simulink model "E11_implementation"  (R2017a)
settings: Solver=VariableStepAuto  StartTime=0.0  StopTime=100  RelTol=1e-3
InitFcn:
  | clear
  | E_param
undefined symbols (not defined in the file or in its folder): E_animation
settings Model: Creator=Mat Haskell  LastModifiedBy=Mat Haskell

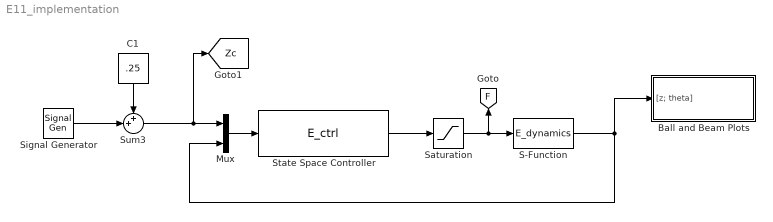
== system E11_implementation ==
  Ball and Beam Plots : Subsystem
  C1 : Constant  Value=.25
  Mux : Mux  Inputs=2
  S-Function : S-Function  FunctionName=E_dynamics  Parameters=P  SFunctionDeploymentMode=off  EnableBusSupport=off
  Saturation : Saturate  UpperLimit=15  LowerLimit=0
  Signal Generator : SignalGenerator  WaveForm=square  Amplitude=.125  Frequency=.05
  State Space Controller : MATLABFcn  MATLABFcn=E_ctrl
  Sum3 : Sum  Inputs=++|
  tag scope: F=global, Zc=global
  wires:
  Sum3/1 -> [Zc], Mux/1
  Saturation/1 -> S-Function/1, [F]
  S-Function/1 -> Mux/2, Ball and Beam Plots/1("[z; theta]")
  C1/1 -> Sum3/1
  Signal Generator/1 -> Sum3/2
  State Space Controller/1 -> Saturation/1
  Mux/1 -> State Space Controller/1

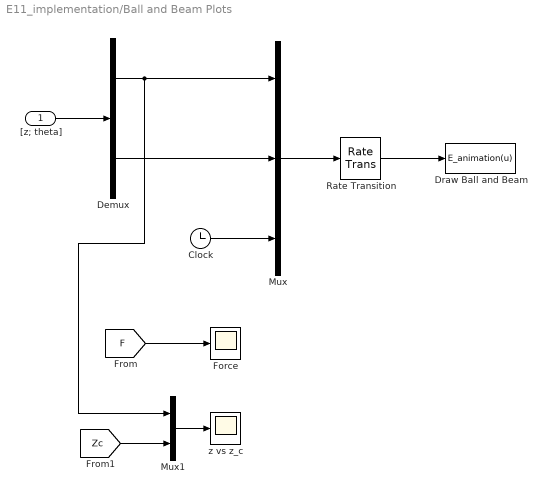
== system E11_implementation/Ball and Beam Plots ==
  "[z; theta]" : Inport
  Clock : Clock
  Demux : Demux  Outputs=2
  Draw Ball and Beam : MATLABFcn  MATLABFcn=E_animation(u)  OutputDimensions=0
  Force : Scope
  Mux : Mux  Inputs=3
  Mux1 : Mux  Inputs=2
  Rate Transition : RateTransition  OutPortSampleTime=P.t_plot
  z vs z_c : Scope
  wires:
  "[z; theta]"/1 -> Demux/1
  Rate Transition/1 -> Draw Ball and Beam/1
  Mux/1 -> Rate Transition/1
  Clock/1 -> Mux/3
  Demux/1 -> Mux1/1, Mux/1
  Demux/2 -> Mux/2
  [F] -> Force/1
  Mux1/1 -> z vs z_c/1
  [Zc] -> Mux1/2
